simulink library "Electrical_to_Thermal_gen"  (R2016a)
settings: Solver=ode1  StartTime=0.0  StopTime=Inf  FixedStep=0.001  RelTol=1e-3
undefined symbols (not defined in the file): brakeresistors_Brc_Coolent_Inlet_Temp, brakeresistors_BRC_InvStError, brakeresistors_Brc_Powerderating, brakeresistors_BRCMaxPwr, brakeresistors_NumBrkResistors, Brc_Coolent_Inlet_Temp, BRC_InvStError, Brc_Powerderating, drvEmot_InvStEnable, drvEmot_InvStError, drvEmot_InvStInit, drvEmot_InvStReady, InvStEnable, InvStError, InvStInit, InvStReady, NumBrkResistors
libraries: simulink x3, Electrical_to_Thermal_gen x1
settings Model: Creator=SAHOPRA  LastModifiedBy=krishs1
settings DataIOCC: LimitDataPoints=on  SaveFormat=Array
settings OptimizationCC: BlockReduction=off  OptimizeBlockIOStorage=off  BufferReuse=off  GlobalBufferReuse=off  ExpressionFolding=off  ExpressionDepthLimit=2147483647  LocalBlockOutputs=off
settings DebuggingCC: UnderspecifiedInitializationDetection=Classic  MergeDetectMultiDrivingBlocksExec=none  SolverPrmCheckMsg=warning  StateNameClashWarn=warning
settings HardwareCC: ProdBitPerPointer=32  ProdLargestAtomicFloat=None  ProdIntDivRoundTo=Undefined  ProdEndianess=Unspecified  ProdWordSize=32  ProdHWDeviceType=32-bit Generic
settings ModelReferenceCC: PropagateSignalLabelsOutOfModel=off
settings RTWCC: SystemTargetFile=rti1005.tlc  MakeCommand=make_rti  TemplateMakefile=rti1005.tmf  Description=dSPACE DS1005 Hardware Platform
settings STFCustomTargetCC: ModelReferenceCompliant=off  GeneratePreprocessorConditionals=Disable all  CombineOutputUpdateFcns=on  MatFileLogging=on  MATLABClassNameForMDSCustomization=Simulink.SoftwareTarget.TargetSpecificTriggerConfigurationBase  CPPClassGenCompliant=on  GRTInterface=off  SystemTargetFile=rti1005.tlc
settings ConfigComp: CovModelRefEnable=Off

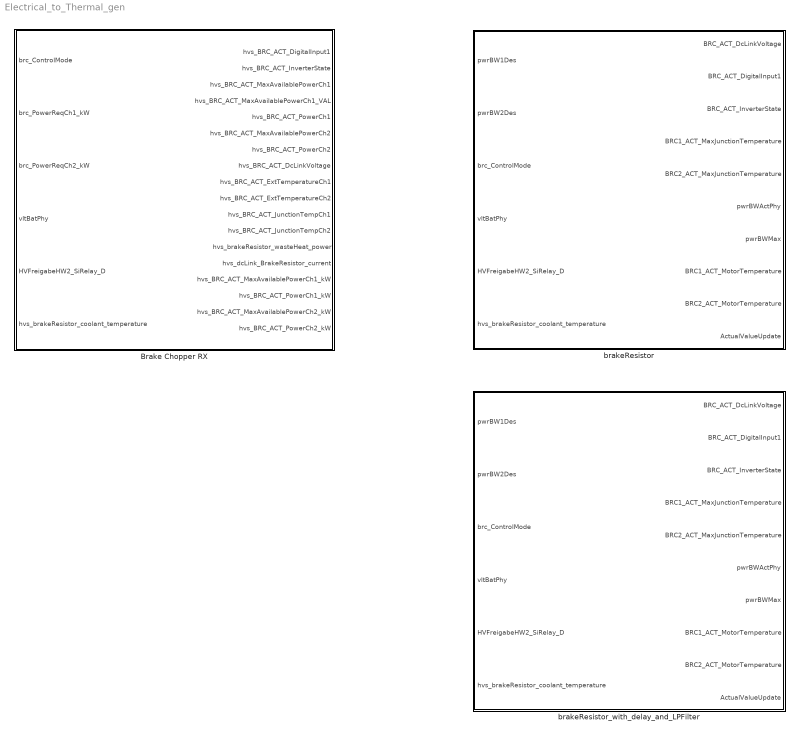
== system Electrical_to_Thermal_gen ==
  Brake Chopper RX : Subsystem
  brakeResistor : Subsystem
  brakeResistor_with_delay_and_LPFilter : Subsystem

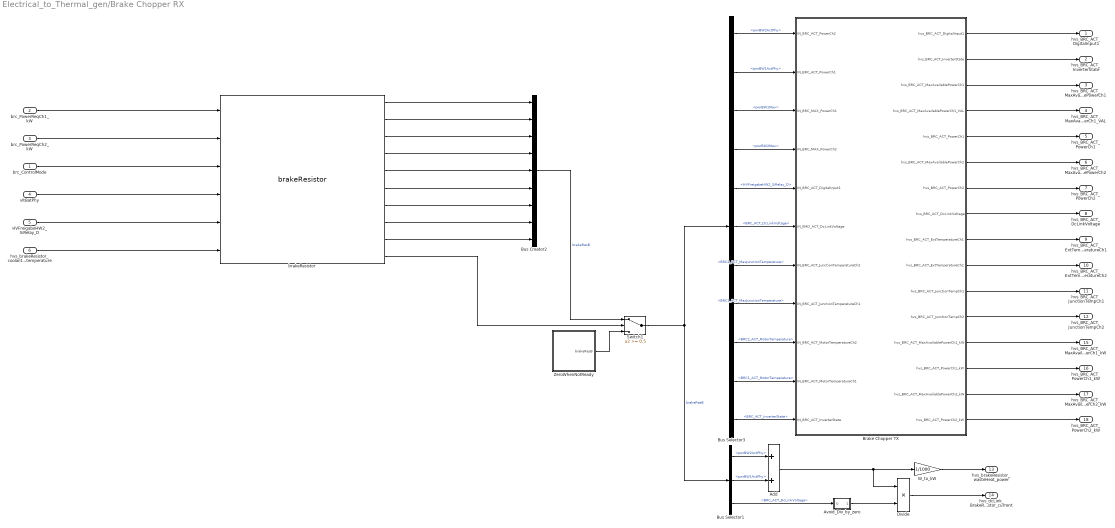
== system Electrical_to_Thermal_gen/Brake Chopper RX ==
  brc_ControlMode : Inport
  brc_PowerReqCh1_kW : Inport  Port=2
  brc_PowerReqCh2_kW : Inport  Port=3
  vltBatPhy : Inport  Port=4
  HVFreigabeHW2_SiRelay_D : Inport  Port=5
  hvs_brakeResistor_coolant_temperature : Inport  Port=6
  Add : Sum
  Avoid_Div_by_zero : Subsystem
  Brake Chopper TX : Subsystem
  Bus Creator2 : BusCreator  Inputs=9
  Bus Selector1 : BusSelector  OutputSignals=pwrBWActPhy.pwrBW2ActPhy,pwrBWActPhy.pwrBW1ActPhy,BRC_ACT_DcLinkVoltage
  Bus Selector3 : BusSelector  OutputSignals=pwrBWActPhy.pwrBW2ActPhy,pwrBWActPhy.pwrBW1ActPhy,pwrBWMax.pwrBW1Max,pwrBWMax.pwrBW2Max,HVFreigabeHW2_SiRelay_D,BRC_ACT_DcLinkVoltage,BRC2_ACT_MaxJunctionTemperature,BRC1_ACT_MaxJunctionTemperature,BRC2_ACT_MotorTemperature,BRC1_ACT_MotorTemperature,BRC_ACT_InverterState
  Divide : Product  Inputs=**
  Switch1 : Switch  Threshold=0.5
  W_to_kW : Gain  Gain=1/1000
      settings: AttributesFormatString=%<Description>
  ZeroWhenNotReady : Subsystem  TreatAsAtomicUnit=on
  brakeResistor : Electrical_to_Thermal_gen/brakeResistor  SystemSampleTime=-1
  hvs_BRC_ACT_DigitalInput1 : Outport
  hvs_BRC_ACT_InverterState : Outport  Port=2
  hvs_BRC_ACT_MaxAvailablePowerCh1 : Outport  Port=3
  hvs_BRC_ACT_MaxAvailablePowerCh1_VAL : Outport  Port=4
  hvs_BRC_ACT_PowerCh1 : Outport  Port=5
  hvs_BRC_ACT_MaxAvailablePowerCh2 : Outport  Port=6
  hvs_BRC_ACT_PowerCh2 : Outport  Port=7
  hvs_BRC_ACT_DcLinkVoltage : Outport  Port=8
  hvs_BRC_ACT_ExtTemperatureCh1 : Outport  Port=9
  hvs_BRC_ACT_ExtTemperatureCh2 : Outport  Port=10
  hvs_BRC_ACT_JunctionTempCh1 : Outport  Port=11
  hvs_BRC_ACT_JunctionTempCh2 : Outport  Port=12
  hvs_brakeResistor_wasteHeat_power : Outport  Port=13
  hvs_dcLink_BrakeResistor_current : Outport  Port=14
  hvs_BRC_ACT_MaxAvailablePowerCh1_kW : Outport  Port=15
  hvs_BRC_ACT_PowerCh1_kW : Outport  Port=16
  hvs_BRC_ACT_MaxAvailablePowerCh2_kW : Outport  Port=17
  hvs_BRC_ACT_PowerCh2_kW : Outport  Port=18
  wires:
  W_to_kW/1 -> hvs_brakeResistor_wasteHeat_power/1
  hvs_brakeResistor_coolant_temperature/1 -> brakeResistor/6
  Divide/1 -> hvs_dcLink_BrakeResistor_current/1
  Avoid_Div_by_zero/1(1/U) -> Divide/2
  Bus Selector1/3 -> Avoid_Div_by_zero/1(U)  "<BRC_ACT_DcLinkVoltage>"
  Add/1 -> W_to_kW/1, Divide/1
  Bus Selector1/2 -> Add/2  "<pwrBW1ActPhy>"
  Bus Selector1/1 -> Add/1  "<pwrBW2ActPhy>"
  HVFreigabeHW2_SiRelay_D/1 -> brakeResistor/5
  Brake Chopper TX/12(hvs_BRC_ACT_JunctionTempCh2) -> hvs_BRC_ACT_JunctionTempCh2/1
  Brake Chopper TX/11(hvs_BRC_ACT_JunctionTempCh1) -> hvs_BRC_ACT_JunctionTempCh1/1
  Brake Chopper TX/10(hvs_BRC_ACT_ExtTemperatureCh2) -> hvs_BRC_ACT_ExtTemperatureCh2/1
  Brake Chopper TX/9(hvs_BRC_ACT_ExtTemperatureCh1) -> hvs_BRC_ACT_ExtTemperatureCh1/1
  Brake Chopper TX/8(hvs_BRC_ACT_DcLinkVoltage) -> hvs_BRC_ACT_DcLinkVoltage/1
  Brake Chopper TX/7(hvs_BRC_ACT_PowerCh2) -> hvs_BRC_ACT_PowerCh2/1
  Brake Chopper TX/6(hvs_BRC_ACT_MaxAvailablePowerCh2) -> hvs_BRC_ACT_MaxAvailablePowerCh2/1
  Brake Chopper TX/5(hvs_BRC_ACT_PowerCh1) -> hvs_BRC_ACT_PowerCh1/1
  Brake Chopper TX/4(hvs_BRC_ACT_MaxAvailablePowerCh1_VAL) -> hvs_BRC_ACT_MaxAvailablePowerCh1_VAL/1
  Brake Chopper TX/3(hvs_BRC_ACT_MaxAvailablePowerCh1) -> hvs_BRC_ACT_MaxAvailablePowerCh1/1
  Brake Chopper TX/2(hvs_BRC_ACT_InverterState) -> hvs_BRC_ACT_InverterState/1
  Brake Chopper TX/1(hvs_BRC_ACT_DigitalInput1) -> hvs_BRC_ACT_DigitalInput1/1
  Bus Selector3/3 -> Brake Chopper TX/3(IN_BRC_MAX_PowerCh1)  "<pwrBW1Max>"
  Bus Selector3/5 -> Brake Chopper TX/5(IN_BRC_ACT_DigitalInput1)  "<HVFreigabeHW2_SiRelay_D>"
  Bus Selector3/4 -> Brake Chopper TX/4(IN_BRC_MAX_PowerCh2)  "<pwrBW2Max>"
  Bus Selector3/1 -> Brake Chopper TX/1(IN_BRC_ACT_PowerCh2)  "<pwrBW2ActPhy>"
  Bus Selector3/2 -> Brake Chopper TX/2(IN_BRC_ACT_PowerCh1)  "<pwrBW1ActPhy>"
  Bus Selector3/6 -> Brake Chopper TX/6(IN_EMD_ACT_DcLinkVoltage)  "<BRC_ACT_DcLinkVoltage>"
  Bus Selector3/7 -> Brake Chopper TX/7(IN_BRC_ACT_JunctionTemperatureCh2)  "<BRC2_ACT_MaxJunctionTemperature>"
  Bus Selector3/8 -> Brake Chopper TX/8(IN_BRC_ACT_JunctionTemperatureCh1)  "<BRC1_ACT_MaxJunctionTemperature>"
  Bus Selector3/9 -> Brake Chopper TX/9(IN_BRC_ACT_MotorTemperatureCh2)  "<BRC2_ACT_MotorTemperature>"
  Bus Selector3/10 -> Brake Chopper TX/10(IN_BRC_ACT_MotorTemperatureCh1)  "<BRC1_ACT_MotorTemperature>"
  Bus Selector3/11 -> Brake Chopper TX/11(IN_BRC_ACT_InverterState)  "<BRC_ACT_InverterState>"
  vltBatPhy/1 -> brakeResistor/4
  brc_PowerReqCh2_kW/1 -> brakeResistor/2
  brc_PowerReqCh1_kW/1 -> brakeResistor/1
  brc_ControlMode/1 -> brakeResistor/3
  Bus Creator2/1 -> Switch1/1  "brakeResB"
  Switch1/1 -> Bus Selector3/1, Bus Selector1/1  "brakeResB"
  ZeroWhenNotReady/1(brakeResB) -> Switch1/3
  brakeResistor/6 -> Bus Creator2/6
  brakeResistor/7 -> Bus Creator2/7
  brakeResistor/8 -> Bus Creator2/8
  brakeResistor/5 -> Bus Creator2/5
  brakeResistor/4 -> Bus Creator2/4
  brakeResistor/3 -> Bus Creator2/3
  brakeResistor/2 -> Bus Creator2/2
  brakeResistor/1 -> Bus Creator2/1
  brakeResistor/9 -> Bus Creator2/9
  Brake Chopper TX/13(hvs_BRC_ACT_MaxAvailablePowerCh1_kW) -> hvs_BRC_ACT_MaxAvailablePowerCh1_kW/1
  Brake Chopper TX/14(hvs_BRC_ACT_PowerCh1_kW) -> hvs_BRC_ACT_PowerCh1_kW/1
  Brake Chopper TX/15(hvs_BRC_ACT_MaxAvailablePowerCh2_kW) -> hvs_BRC_ACT_MaxAvailablePowerCh2_kW/1
  Brake Chopper TX/16(hvs_BRC_ACT_PowerCh2_kW) -> hvs_BRC_ACT_PowerCh2_kW/1
  brakeResistor/10 -> Switch1/2

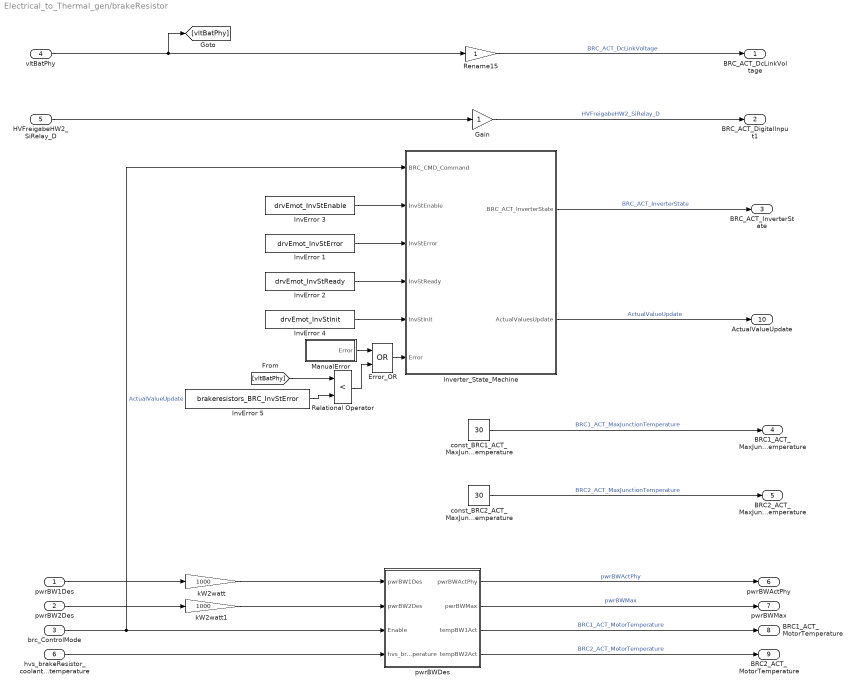
== system Electrical_to_Thermal_gen/brakeResistor ==
  pwrBW1Des : Inport
  pwrBW2Des : Inport  Port=2
  brc_ControlMode : Inport  Port=3
  vltBatPhy : Inport  Port=4
  HVFreigabeHW2_SiRelay_D : Inport  Port=5
  hvs_brakeResistor_coolant_temperature : Inport  Port=6
  Error_OR : Logic  Operator=OR  AllPortsSameDT=off  OutDataTypeStr=boolean
  Gain : Gain
  InvError 1 : Constant  Value=drvEmot_InvStError
  InvError 2 : Constant  Value=drvEmot_InvStReady
  InvError 3 : Constant  Value=drvEmot_InvStEnable
  InvError 4 : Constant  Value=drvEmot_InvStInit
  InvError 5 : Constant  Value=brakeresistors_BRC_InvStError
  Inverter_State_Machine : Stateflow chart  TreatAsAtomicUnit=on
  ManualError : Subsystem  TreatAsAtomicUnit=on
  Relational Operator : RelationalOperator  Operator=<  OutDataTypeStr=boolean
  Rename15 : Gain
  const_BRC1_ACT_MaxJunctionTemperature : Constant  Value=30
  const_BRC2_ACT_MaxJunctionTemperature : Constant  Value=30
  kW2watt : Gain  Gain=1000
  kW2watt1 : Gain  Gain=1000
  "pwrBWDes " : Subsystem
  BRC_ACT_DcLinkVoltage : Outport
  " BRC_ACT_DigitalInput1" : Outport  Port=2
  BRC_ACT_InverterState : Outport  Port=3
  BRC1_ACT_MaxJunctionTemperature : Outport  Port=4
  BRC2_ACT_MaxJunctionTemperature : Outport  Port=5
  pwrBWActPhy : Outport  Port=6
  pwrBWMax : Outport  Port=7
  BRC1_ACT_MotorTemperature : Outport  Port=8
  BRC2_ACT_MotorTemperature : Outport  Port=9
  ActualValueUpdate : Outport  Port=10
  wires:
  kW2watt1/1 -> "pwrBWDes "/2(pwrBW2Des)
  kW2watt/1 -> "pwrBWDes "/1(pwrBW1Des)
  pwrBW2Des/1 -> kW2watt1/1
  pwrBW1Des/1 -> kW2watt/1
  HVFreigabeHW2_SiRelay_D/1 -> Gain/1
  brc_ControlMode/1 -> "pwrBWDes "/3(Enable), Inverter_State_Machine/1(BRC_CMD_Command)  "ActualValueUpdate"
  Rename15/1 -> BRC_ACT_DcLinkVoltage/1  "BRC_ACT_DcLinkVoltage"
  "pwrBWDes "/4(tempBW2Act) -> BRC2_ACT_MotorTemperature/1  "BRC2_ACT_MotorTemperature"
  "pwrBWDes "/3(tempBW1Act) -> BRC1_ACT_MotorTemperature/1  "BRC1_ACT_MotorTemperature"
  Gain/1 -> " BRC_ACT_DigitalInput1"/1  "HVFreigabeHW2_SiRelay_D"
  const_BRC2_ACT_MaxJunctionTemperature/1 -> BRC2_ACT_MaxJunctionTemperature/1  "BRC2_ACT_MaxJunctionTemperature"
  const_BRC1_ACT_MaxJunctionTemperature/1 -> BRC1_ACT_MaxJunctionTemperature/1  "BRC1_ACT_MaxJunctionTemperature"
  "pwrBWDes "/2(pwrBWMax) -> pwrBWMax/1  "pwrBWMax"
  "pwrBWDes "/1(pwrBWActPhy) -> pwrBWActPhy/1  "pwrBWActPhy"
  hvs_brakeResistor_coolant_temperature/1 -> "pwrBWDes "/4(hvs_brakeResistor_coolant_temperature)
  InvError 1/1 -> Inverter_State_Machine/3(InvStError)
  InvError 2/1 -> Inverter_State_Machine/4(InvStReady)
  InvError 3/1 -> Inverter_State_Machine/2(InvStEnable)
  InvError 4/1 -> Inverter_State_Machine/5(InvStInit)
  Inverter_State_Machine/1(BRC_ACT_InverterState) -> BRC_ACT_InverterState/1  "BRC_ACT_InverterState"
  Error_OR/1 -> Inverter_State_Machine/6(Error)
  Inverter_State_Machine/2(ActualValuesUpdate) -> ActualValueUpdate/1  "ActualValueUpdate"
  ManualError/1(Error) -> Error_OR/1
  Relational Operator/1 -> Error_OR/2
  InvError 5/1 -> Relational Operator/2
  vltBatPhy/1 -> [vltBatPhy], Rename15/1
  [vltBatPhy] -> Relational Operator/1

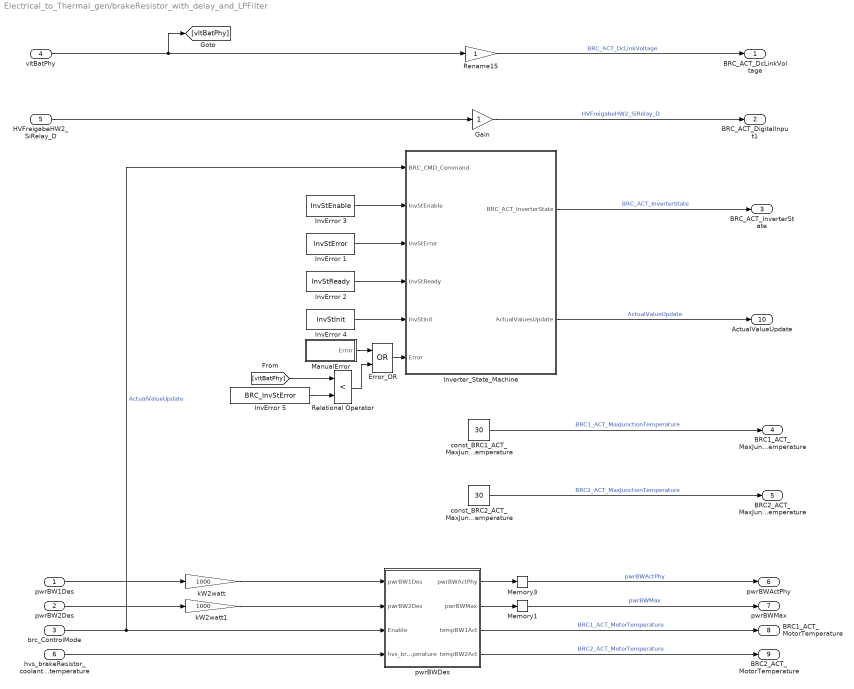
== system Electrical_to_Thermal_gen/brakeResistor_with_delay_and_LPFilter ==
  pwrBW1Des : Inport
  pwrBW2Des : Inport  Port=2
  brc_ControlMode : Inport  Port=3
  vltBatPhy : Inport  Port=4
  HVFreigabeHW2_SiRelay_D : Inport  Port=5
  hvs_brakeResistor_coolant_temperature : Inport  Port=6
  Error_OR : Logic  Operator=OR  AllPortsSameDT=off  OutDataTypeStr=boolean
  Gain : Gain
  InvError 1 : Constant  Value=InvStError
  InvError 2 : Constant  Value=InvStReady
  InvError 3 : Constant  Value=InvStEnable
  InvError 4 : Constant  Value=InvStInit
  InvError 5 : Constant  Value=BRC_InvStError
  Inverter_State_Machine : Stateflow chart  TreatAsAtomicUnit=on
  ManualError : Subsystem  TreatAsAtomicUnit=on
  Memory1 : Memory
  Memory3 : Memory
  Relational Operator : RelationalOperator  Operator=<  OutDataTypeStr=boolean
  Rename15 : Gain
  const_BRC1_ACT_MaxJunctionTemperature : Constant  Value=30
  const_BRC2_ACT_MaxJunctionTemperature : Constant  Value=30
  kW2watt : Gain  Gain=1000
  kW2watt1 : Gain  Gain=1000
  "pwrBWDes " : Subsystem
  BRC_ACT_DcLinkVoltage : Outport
  " BRC_ACT_DigitalInput1" : Outport  Port=2
  BRC_ACT_InverterState : Outport  Port=3
  BRC1_ACT_MaxJunctionTemperature : Outport  Port=4
  BRC2_ACT_MaxJunctionTemperature : Outport  Port=5
  pwrBWActPhy : Outport  Port=6
  pwrBWMax : Outport  Port=7
  BRC1_ACT_MotorTemperature : Outport  Port=8
  BRC2_ACT_MotorTemperature : Outport  Port=9
  ActualValueUpdate : Outport  Port=10
  wires:
  kW2watt1/1 -> "pwrBWDes "/2(pwrBW2Des)
  kW2watt/1 -> "pwrBWDes "/1(pwrBW1Des)
  pwrBW2Des/1 -> kW2watt1/1
  pwrBW1Des/1 -> kW2watt/1
  HVFreigabeHW2_SiRelay_D/1 -> Gain/1
  brc_ControlMode/1 -> "pwrBWDes "/3(Enable), Inverter_State_Machine/1(BRC_CMD_Command)  "ActualValueUpdate"
  Rename15/1 -> BRC_ACT_DcLinkVoltage/1  "BRC_ACT_DcLinkVoltage"
  "pwrBWDes "/4(tempBW2Act) -> BRC2_ACT_MotorTemperature/1  "BRC2_ACT_MotorTemperature"
  "pwrBWDes "/3(tempBW1Act) -> BRC1_ACT_MotorTemperature/1  "BRC1_ACT_MotorTemperature"
  Gain/1 -> " BRC_ACT_DigitalInput1"/1  "HVFreigabeHW2_SiRelay_D"
  const_BRC2_ACT_MaxJunctionTemperature/1 -> BRC2_ACT_MaxJunctionTemperature/1  "BRC2_ACT_MaxJunctionTemperature"
  const_BRC1_ACT_MaxJunctionTemperature/1 -> BRC1_ACT_MaxJunctionTemperature/1  "BRC1_ACT_MaxJunctionTemperature"
  Memory1/1 -> pwrBWMax/1  "pwrBWMax"
  "pwrBWDes "/2(pwrBWMax) -> Memory1/1
  Memory3/1 -> pwrBWActPhy/1  "pwrBWActPhy"
  "pwrBWDes "/1(pwrBWActPhy) -> Memory3/1
  hvs_brakeResistor_coolant_temperature/1 -> "pwrBWDes "/4(hvs_brakeResistor_coolant_temperature)
  InvError 1/1 -> Inverter_State_Machine/3(InvStError)
  InvError 2/1 -> Inverter_State_Machine/4(InvStReady)
  InvError 3/1 -> Inverter_State_Machine/2(InvStEnable)
  InvError 4/1 -> Inverter_State_Machine/5(InvStInit)
  Inverter_State_Machine/1(BRC_ACT_InverterState) -> BRC_ACT_InverterState/1  "BRC_ACT_InverterState"
  Error_OR/1 -> Inverter_State_Machine/6(Error)
  Inverter_State_Machine/2(ActualValuesUpdate) -> ActualValueUpdate/1  "ActualValueUpdate"
  ManualError/1(Error) -> Error_OR/1
  Relational Operator/1 -> Error_OR/2
  InvError 5/1 -> Relational Operator/2
  vltBatPhy/1 -> [vltBatPhy], Rename15/1
  [vltBatPhy] -> Relational Operator/1

== system Electrical_to_Thermal_gen/Brake Chopper RX/Avoid_Div_by_zero ==
  U : Inport
  Constant : Constant  Value=10^-6
  Divide : Product  Inputs=/*
  Math Function : Math  Operator=square  SaturateOnIntegerOverflow=on
  Sum : Sum  Inputs=++|
  1/U : Outport
  wires:
  U/1 -> Sum/2
  Constant/1 -> Sum/1
  Sum/1 -> Math Function/1, Divide/2
  Math Function/1 -> Divide/1
  Divide/1 -> 1/U/1

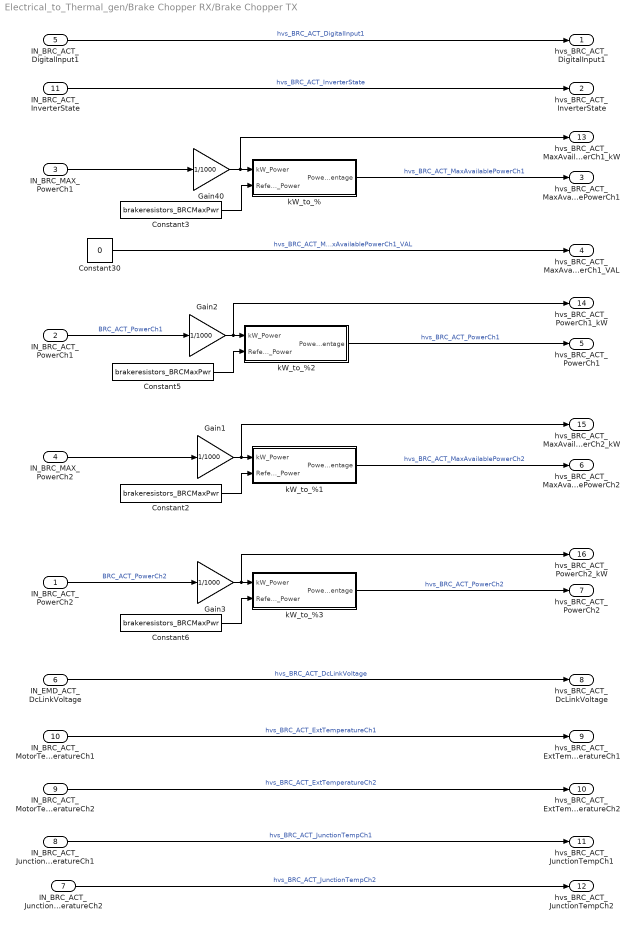
== system Electrical_to_Thermal_gen/Brake Chopper RX/Brake Chopper TX ==
  IN_BRC_ACT_PowerCh2 : Inport
  IN_BRC_ACT_PowerCh1 : Inport  Port=2
  IN_BRC_MAX_PowerCh1 : Inport  Port=3
  IN_BRC_MAX_PowerCh2 : Inport  Port=4
  IN_BRC_ACT_DigitalInput1 : Inport  Port=5
  IN_EMD_ACT_DcLinkVoltage : Inport  Port=6
  IN_BRC_ACT_JunctionTemperatureCh2 : Inport  Port=7
  IN_BRC_ACT_JunctionTemperatureCh1 : Inport  Port=8
  IN_BRC_ACT_MotorTemperatureCh2 : Inport  Port=9
  IN_BRC_ACT_MotorTemperatureCh1 : Inport  Port=10
  IN_BRC_ACT_InverterState : Inport  Port=11
  Constant{2..3,5..6} (4 alike) : Constant  Value=brakeresistors_BRCMaxPwr
  Constant30 : Constant  Value=0
  Gain{1..3,40} (4 alike) : Gain  Gain=1/1000
  kW_to_% : Subsystem
  kW_to_%1 : Subsystem
  kW_to_%2 : Subsystem
  kW_to_%3 : Subsystem
  hvs_BRC_ACT_DigitalInput1 : Outport
  hvs_BRC_ACT_InverterState : Outport  Port=2
  hvs_BRC_ACT_MaxAvailablePowerCh1 : Outport  Port=3
  hvs_BRC_ACT_MaxAvailablePowerCh1_VAL : Outport  Port=4
  hvs_BRC_ACT_PowerCh1 : Outport  Port=5
  hvs_BRC_ACT_MaxAvailablePowerCh2 : Outport  Port=6
  hvs_BRC_ACT_PowerCh2 : Outport  Port=7
  hvs_BRC_ACT_DcLinkVoltage : Outport  Port=8
  hvs_BRC_ACT_ExtTemperatureCh1 : Outport  Port=9
  hvs_BRC_ACT_ExtTemperatureCh2 : Outport  Port=10
  hvs_BRC_ACT_JunctionTempCh1 : Outport  Port=11
  hvs_BRC_ACT_JunctionTempCh2 : Outport  Port=12
  hvs_BRC_ACT_MaxAvailablePowerCh1_kW : Outport  Port=13
  hvs_BRC_ACT_PowerCh1_kW : Outport  Port=14
  hvs_BRC_ACT_MaxAvailablePowerCh2_kW : Outport  Port=15
  hvs_BRC_ACT_PowerCh2_kW : Outport  Port=16
  wires:
  Constant30/1 -> hvs_BRC_ACT_MaxAvailablePowerCh1_VAL/1  "hvs_BRC_ACT_MaxAvailablePowerCh1_VAL"
  Constant6/1 -> kW_to_%3/2(Reference_Power)
  Gain3/1 -> hvs_BRC_ACT_PowerCh2_kW/1, kW_to_%3/1(kW_Power)
  IN_BRC_ACT_PowerCh2/1 -> Gain3/1  "BRC_ACT_PowerCh2"
  Constant5/1 -> kW_to_%2/2(Reference_Power)
  Gain2/1 -> hvs_BRC_ACT_PowerCh1_kW/1, kW_to_%2/1(kW_Power)
  IN_BRC_ACT_PowerCh1/1 -> Gain2/1  "BRC_ACT_PowerCh1"
  Gain1/1 -> hvs_BRC_ACT_MaxAvailablePowerCh2_kW/1, kW_to_%1/1(kW_Power)
  Constant2/1 -> kW_to_%1/2(Reference_Power)
  Constant3/1 -> kW_to_%/2(Reference_Power)
  Gain40/1 -> hvs_BRC_ACT_MaxAvailablePowerCh1_kW/1, kW_to_%/1(kW_Power)
  kW_to_%1/1(Power_Percentage) -> hvs_BRC_ACT_MaxAvailablePowerCh2/1  "hvs_BRC_ACT_MaxAvailablePowerCh2"
  IN_BRC_MAX_PowerCh2/1 -> Gain1/1
  kW_to_%/1(Power_Percentage) -> hvs_BRC_ACT_MaxAvailablePowerCh1/1  "hvs_BRC_ACT_MaxAvailablePowerCh1"
  IN_BRC_MAX_PowerCh1/1 -> Gain40/1
  IN_BRC_ACT_DigitalInput1/1 -> hvs_BRC_ACT_DigitalInput1/1  "hvs_BRC_ACT_DigitalInput1"
  IN_BRC_ACT_JunctionTemperatureCh1/1 -> hvs_BRC_ACT_JunctionTempCh1/1  "hvs_BRC_ACT_JunctionTempCh1"
  IN_BRC_ACT_JunctionTemperatureCh2/1 -> hvs_BRC_ACT_JunctionTempCh2/1  "hvs_BRC_ACT_JunctionTempCh2"
  IN_EMD_ACT_DcLinkVoltage/1 -> hvs_BRC_ACT_DcLinkVoltage/1  "hvs_BRC_ACT_DcLinkVoltage"
  kW_to_%3/1(Power_Percentage) -> hvs_BRC_ACT_PowerCh2/1  "hvs_BRC_ACT_PowerCh2"
  IN_BRC_ACT_MotorTemperatureCh2/1 -> hvs_BRC_ACT_ExtTemperatureCh2/1  "hvs_BRC_ACT_ExtTemperatureCh2"
  kW_to_%2/1(Power_Percentage) -> hvs_BRC_ACT_PowerCh1/1  "hvs_BRC_ACT_PowerCh1"
  IN_BRC_ACT_MotorTemperatureCh1/1 -> hvs_BRC_ACT_ExtTemperatureCh1/1  "hvs_BRC_ACT_ExtTemperatureCh1"
  IN_BRC_ACT_InverterState/1 -> hvs_BRC_ACT_InverterState/1  "hvs_BRC_ACT_InverterState"

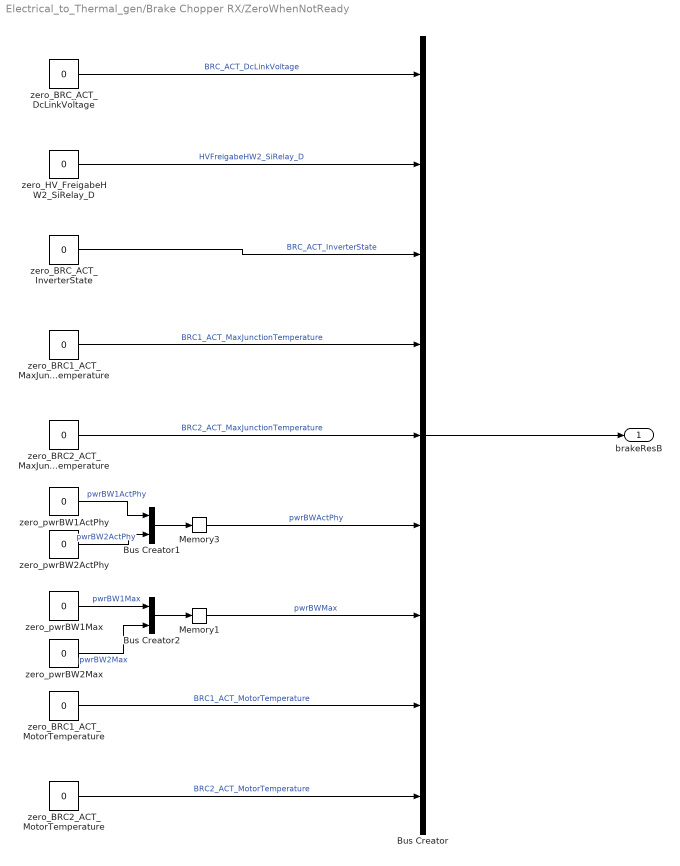
== system Electrical_to_Thermal_gen/Brake Chopper RX/ZeroWhenNotReady ==
  Bus Creator : BusCreator  Inputs=9
  Bus Creator1 : BusCreator  Inputs=2
  Bus Creator2 : BusCreator  Inputs=2
  Memory1 : Memory  InheritSampleTime=on
  Memory3 : Memory  InheritSampleTime=on
  zero_BRC1_ACT_MaxJunctionTemperature : Constant  Value=0
  zero_BRC1_ACT_MotorTemperature : Constant  Value=0
  zero_BRC2_ACT_MaxJunctionTemperature : Constant  Value=0
  zero_BRC2_ACT_MotorTemperature : Constant  Value=0
  zero_BRC_ACT_DcLinkVoltage : Constant  Value=0
  zero_BRC_ACT_InverterState : Constant  Value=0
  zero_HV_FreigabeHW2_SiRelay_D : Constant  Value=0
  zero_pwrBW1ActPhy : Constant  Value=0
  zero_pwrBW1Max : Constant  Value=0
  zero_pwrBW2ActPhy : Constant  Value=0
  zero_pwrBW2Max : Constant  Value=0
  brakeResB : Outport
  wires:
  zero_HV_FreigabeHW2_SiRelay_D/1 -> Bus Creator/2  "HVFreigabeHW2_SiRelay_D"
  zero_BRC_ACT_InverterState/1 -> Bus Creator/3  "BRC_ACT_InverterState"
  zero_BRC1_ACT_MaxJunctionTemperature/1 -> Bus Creator/4  "BRC1_ACT_MaxJunctionTemperature"
  zero_BRC2_ACT_MaxJunctionTemperature/1 -> Bus Creator/5  "BRC2_ACT_MaxJunctionTemperature"
  Memory3/1 -> Bus Creator/6  "pwrBWActPhy"
  Memory1/1 -> Bus Creator/7  "pwrBWMax"
  Bus Creator1/1 -> Memory3/1
  zero_pwrBW1ActPhy/1 -> Bus Creator1/1  "pwrBW1ActPhy"
  zero_pwrBW2ActPhy/1 -> Bus Creator1/2  "pwrBW2ActPhy"
  Bus Creator2/1 -> Memory1/1
  zero_pwrBW1Max/1 -> Bus Creator2/1  "pwrBW1Max"
  zero_pwrBW2Max/1 -> Bus Creator2/2  "pwrBW2Max"
  Bus Creator/1 -> brakeResB/1
  zero_BRC_ACT_DcLinkVoltage/1 -> Bus Creator/1  "BRC_ACT_DcLinkVoltage"
  zero_BRC2_ACT_MotorTemperature/1 -> Bus Creator/9  "BRC2_ACT_MotorTemperature"
  zero_BRC1_ACT_MotorTemperature/1 -> Bus Creator/8  "BRC1_ACT_MotorTemperature"

== system Electrical_to_Thermal_gen/brakeResistor/ManualError ==
  ErrorSwitch : ManualSwitch
  InvError : Constant
  NoError : Constant  Value=0
  Error : Outport
  wires:
  NoError/1 -> ErrorSwitch/1
  InvError/1 -> ErrorSwitch/2
  ErrorSwitch/1 -> Error/1

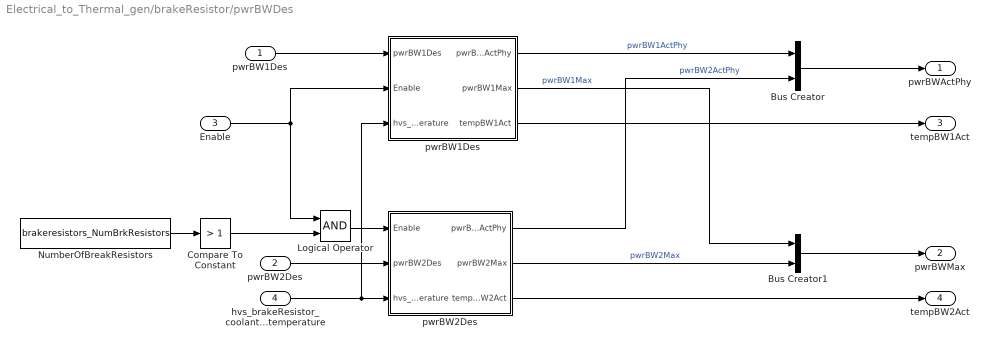
== system Electrical_to_Thermal_gen/brakeResistor/pwrBWDes  ==
  pwrBW1Des : Inport
  pwrBW2Des : Inport  Port=2
  Enable : Inport  Port=3
  hvs_brakeResistor_coolant_temperature : Inport  Port=4
  Bus Creator : BusCreator  Inputs=2
  Bus Creator1 : BusCreator  Inputs=2
  Compare To Constant : simulink/Logic and Bit Operations/Compare To Constant  relop=>  const=1  OutDataTypeStr=boolean
  Logical Operator : Logic  AllPortsSameDT=off  OutDataTypeStr=boolean
  NumberOfBreakResistors : Constant  Value=brakeresistors_NumBrkResistors
  "pwrBW1Des " : Subsystem
  "pwrBW2Des " : Subsystem
  pwrBWActPhy : Outport
  pwrBWMax : Outport  Port=2
  tempBW1Act : Outport  Port=3
  tempBW2Act : Outport  Port=4
  wires:
  hvs_brakeResistor_coolant_temperature/1 -> "pwrBW1Des "/3(hvs_brakeResistor_coolant_temperature), "pwrBW2Des "/3(hvs_brakeResistor_coolant_temperature)
  "pwrBW2Des "/3(tempBW2Act) -> tempBW2Act/1
  "pwrBW1Des "/3(tempBW1Act) -> tempBW1Act/1
  Enable/1 -> Logical Operator/1, "pwrBW1Des "/2(Enable)
  "pwrBW2Des "/2(pwrBW2Max) -> Bus Creator1/2  "pwrBW2Max"
  "pwrBW1Des "/2(pwrBW1Max) -> Bus Creator1/1  "pwrBW1Max"
  "pwrBW1Des "/1(pwrBW1ActPhy) -> Bus Creator/1  "pwrBW1ActPhy"
  Bus Creator1/1 -> pwrBWMax/1
  Bus Creator/1 -> pwrBWActPhy/1
  pwrBW2Des/1 -> "pwrBW2Des "/2(pwrBW2Des)
  pwrBW1Des/1 -> "pwrBW1Des "/1(pwrBW1Des)
  NumberOfBreakResistors/1 -> Compare To Constant/1
  Compare To Constant/1 -> Logical Operator/2
  Logical Operator/1 -> "pwrBW2Des "/1(Enable)
  "pwrBW2Des "/1(pwrBW2ActPhy) -> Bus Creator/2  "pwrBW2ActPhy"

== system Electrical_to_Thermal_gen/brakeResistor_with_delay_and_LPFilter/ManualError ==
  ErrorSwitch : ManualSwitch
  InvError : Constant
  NoError : Constant  Value=0
  Error : Outport
  wires:
  NoError/1 -> ErrorSwitch/1
  InvError/1 -> ErrorSwitch/2
  ErrorSwitch/1 -> Error/1

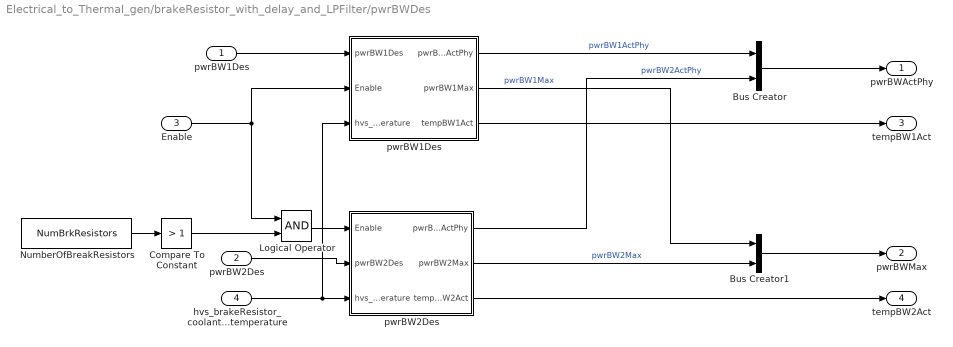
== system Electrical_to_Thermal_gen/brakeResistor_with_delay_and_LPFilter/pwrBWDes  ==
  pwrBW1Des : Inport
  pwrBW2Des : Inport  Port=2
  Enable : Inport  Port=3
  hvs_brakeResistor_coolant_temperature : Inport  Port=4
  Bus Creator : BusCreator  Inputs=2
  Bus Creator1 : BusCreator  Inputs=2
  Compare To Constant : simulink/Logic and Bit Operations/Compare To Constant  relop=>  const=1  OutDataTypeStr=boolean
  Logical Operator : Logic  AllPortsSameDT=off  OutDataTypeStr=boolean
  NumberOfBreakResistors : Constant  Value=NumBrkResistors
  "pwrBW1Des " : Subsystem
  "pwrBW2Des " : Subsystem
  pwrBWActPhy : Outport
  pwrBWMax : Outport  Port=2
  tempBW1Act : Outport  Port=3
  tempBW2Act : Outport  Port=4
  wires:
  hvs_brakeResistor_coolant_temperature/1 -> "pwrBW1Des "/3(hvs_brakeResistor_coolant_temperature), "pwrBW2Des "/3(hvs_brakeResistor_coolant_temperature)
  "pwrBW2Des "/3(tempBW2Act) -> tempBW2Act/1
  "pwrBW1Des "/3(tempBW1Act) -> tempBW1Act/1
  Enable/1 -> Logical Operator/1, "pwrBW1Des "/2(Enable)
  "pwrBW2Des "/2(pwrBW2Max) -> Bus Creator1/2  "pwrBW2Max"
  "pwrBW1Des "/2(pwrBW1Max) -> Bus Creator1/1  "pwrBW1Max"
  "pwrBW1Des "/1(pwrBW1ActPhy) -> Bus Creator/1  "pwrBW1ActPhy"
  Bus Creator1/1 -> pwrBWMax/1
  Bus Creator/1 -> pwrBWActPhy/1
  pwrBW2Des/1 -> "pwrBW2Des "/2(pwrBW2Des)
  pwrBW1Des/1 -> "pwrBW1Des "/1(pwrBW1Des)
  NumberOfBreakResistors/1 -> Compare To Constant/1
  Compare To Constant/1 -> Logical Operator/2
  Logical Operator/1 -> "pwrBW2Des "/1(Enable)
  "pwrBW2Des "/1(pwrBW2ActPhy) -> Bus Creator/2  "pwrBW2ActPhy"

== system Electrical_to_Thermal_gen/Brake Chopper RX/Brake Chopper TX/kW_to_% ==
  kW_Power : Inport
  Reference_Power : Inport  Port=2
  Constant : Constant  Value=100
  Divide1 : Product  Inputs=*/
  Product1 : Product  RndMeth=Zero
  Power_Percentage : Outport
  wires:
  Constant/1 -> Product1/2
  Divide1/1 -> Product1/1
  Reference_Power/1 -> Divide1/2  "Reference_Power"
  Product1/1 -> Power_Percentage/1  "Power_Percentage"
  kW_Power/1 -> Divide1/1  "kW_Power"

== system Electrical_to_Thermal_gen/Brake Chopper RX/Brake Chopper TX/kW_to_%1 ==
  kW_Power : Inport
  Reference_Power : Inport  Port=2
  Constant : Constant  Value=100
  Divide1 : Product  Inputs=*/
  Product1 : Product  RndMeth=Zero
  Power_Percentage : Outport
  wires:
  kW_Power/1 -> Divide1/1  "kW_Power"
  Product1/1 -> Power_Percentage/1  "Power_Percentage"
  Reference_Power/1 -> Divide1/2  "Reference_Power"
  Divide1/1 -> Product1/1
  Constant/1 -> Product1/2

== system Electrical_to_Thermal_gen/Brake Chopper RX/Brake Chopper TX/kW_to_%2 ==
  kW_Power : Inport
  Reference_Power : Inport  Port=2
  Constant : Constant  Value=100
  Divide1 : Product  Inputs=*/
  Product1 : Product  RndMeth=Zero
  Power_Percentage : Outport
  wires:
  Constant/1 -> Product1/2
  Divide1/1 -> Product1/1
  Reference_Power/1 -> Divide1/2  "Reference_Power"
  Product1/1 -> Power_Percentage/1  "Power_Percentage"
  kW_Power/1 -> Divide1/1  "kW_Power"

== system Electrical_to_Thermal_gen/Brake Chopper RX/Brake Chopper TX/kW_to_%3 ==
  kW_Power : Inport
  Reference_Power : Inport  Port=2
  Constant : Constant  Value=100
  Divide1 : Product  Inputs=*/
  Product1 : Product  RndMeth=Zero
  Power_Percentage : Outport
  wires:
  kW_Power/1 -> Divide1/1  "kW_Power"
  Product1/1 -> Power_Percentage/1  "Power_Percentage"
  Reference_Power/1 -> Divide1/2  "Reference_Power"
  Divide1/1 -> Product1/1
  Constant/1 -> Product1/2

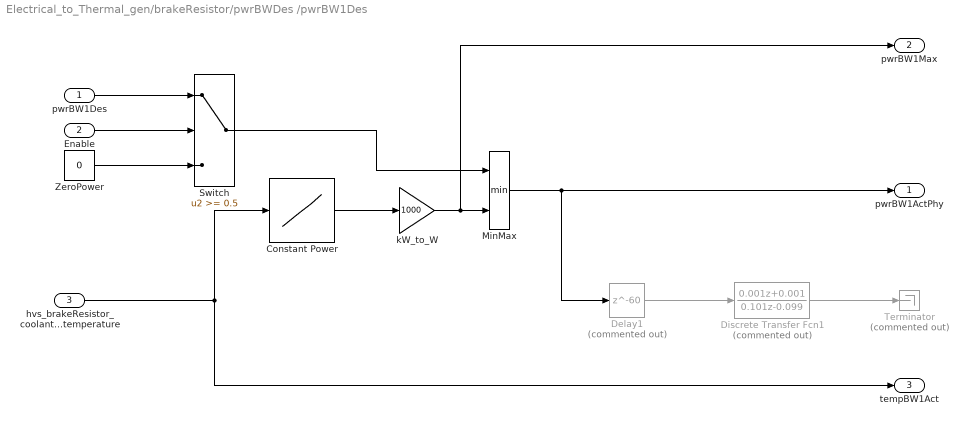
== system Electrical_to_Thermal_gen/brakeResistor/pwrBWDes /pwrBW1Des  ==
  pwrBW1Des : Inport
  Enable : Inport  Port=2
  hvs_brakeResistor_coolant_temperature : Inport  Port=3
  Constant Power : Lookup_n-D  NumberOfTableDimensions=1  BreakpointsForDimension1=brakeresistors_Brc_Coolent_Inlet_Temp  Table=brakeresistors_Brc_Powerderating  ExtrapMethod=Clip  UseLastTableValue=on  RndMeth=Simplest  InputSameDT=on
  Delay1 : Delay  Commented=on  DelayLength=60
  Discrete Transfer Fcn1 : DiscreteTransferFcn  Commented=on  Numerator=[0.001 0.001]  Denominator=[0.101 -0.099]
  MinMax : MinMax  Inputs=2
  Switch : Switch  Threshold=0.5
  Terminator : Terminator  Commented=on
  ZeroPower : Constant  Value=0
  kW_to_W : Gain  Gain=1000
  pwrBW1ActPhy : Outport
  pwrBW1Max : Outport  Port=2
  tempBW1Act : Outport  Port=3
  wires:
  hvs_brakeResistor_coolant_temperature/1 -> Constant Power/1, tempBW1Act/1
  Delay1/1 -> Discrete Transfer Fcn1/1
  MinMax/1 -> pwrBW1ActPhy/1, Delay1/1
  pwrBW1Des/1 -> Switch/1
  ZeroPower/1 -> Switch/3
  Switch/1 -> MinMax/1
  Enable/1 -> Switch/2
  Constant Power/1 -> kW_to_W/1
  Discrete Transfer Fcn1/1 -> Terminator/1
  kW_to_W/1 -> pwrBW1Max/1, MinMax/2

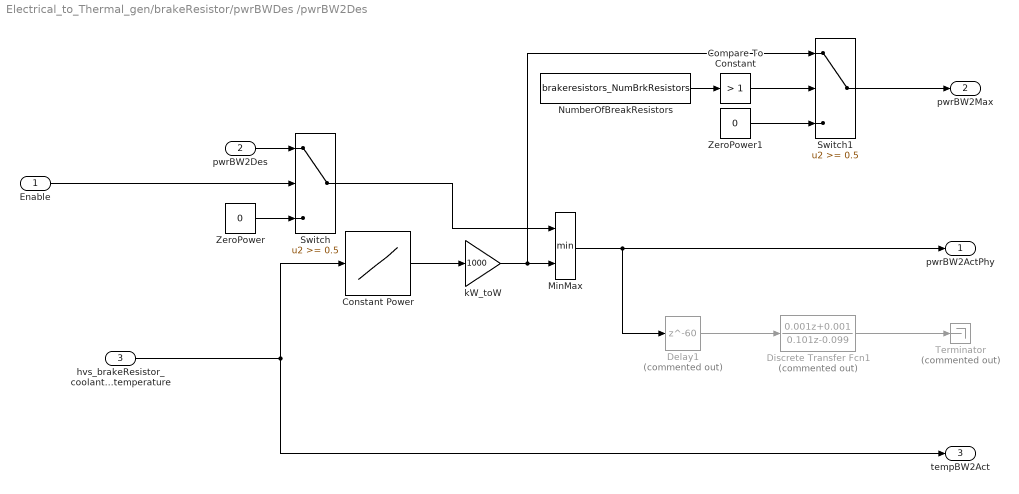
== system Electrical_to_Thermal_gen/brakeResistor/pwrBWDes /pwrBW2Des  ==
  Enable : Inport
  pwrBW2Des : Inport  Port=2
  hvs_brakeResistor_coolant_temperature : Inport  Port=3
  Compare To Constant : simulink/Logic and Bit Operations/Compare To Constant  relop=>  const=1  OutDataTypeStr=boolean
  Constant Power : Lookup_n-D  NumberOfTableDimensions=1  BreakpointsForDimension1=brakeresistors_Brc_Coolent_Inlet_Temp  Table=brakeresistors_Brc_Powerderating  ExtrapMethod=Clip  UseLastTableValue=on  RndMeth=Simplest  InputSameDT=on
  Delay1 : Delay  Commented=on  DelayLength=60
  Discrete Transfer Fcn1 : DiscreteTransferFcn  Commented=on  Numerator=[0.001 0.001]  Denominator=[0.101 -0.099]
  MinMax : MinMax  Inputs=2
  NumberOfBreakResistors : Constant  Value=brakeresistors_NumBrkResistors
  Switch : Switch  Threshold=0.5
  Switch1 : Switch  Threshold=0.5
  Terminator : Terminator  Commented=on
  ZeroPower : Constant  Value=0
  ZeroPower1 : Constant  Value=0
  kW_toW : Gain  Gain=1000
  pwrBW2ActPhy : Outport
  pwrBW2Max : Outport  Port=2
  tempBW2Act : Outport  Port=3
  wires:
  Enable/1 -> Switch/2
  Switch1/1 -> pwrBW2Max/1
  ZeroPower1/1 -> Switch1/3
  hvs_brakeResistor_coolant_temperature/1 -> Constant Power/1, tempBW2Act/1
  Discrete Transfer Fcn1/1 -> Terminator/1
  Delay1/1 -> Discrete Transfer Fcn1/1
  MinMax/1 -> pwrBW2ActPhy/1, Delay1/1
  kW_toW/1 -> MinMax/2, Switch1/1
  pwrBW2Des/1 -> Switch/1
  ZeroPower/1 -> Switch/3
  Switch/1 -> MinMax/1
  Constant Power/1 -> kW_toW/1
  NumberOfBreakResistors/1 -> Compare To Constant/1
  Compare To Constant/1 -> Switch1/2

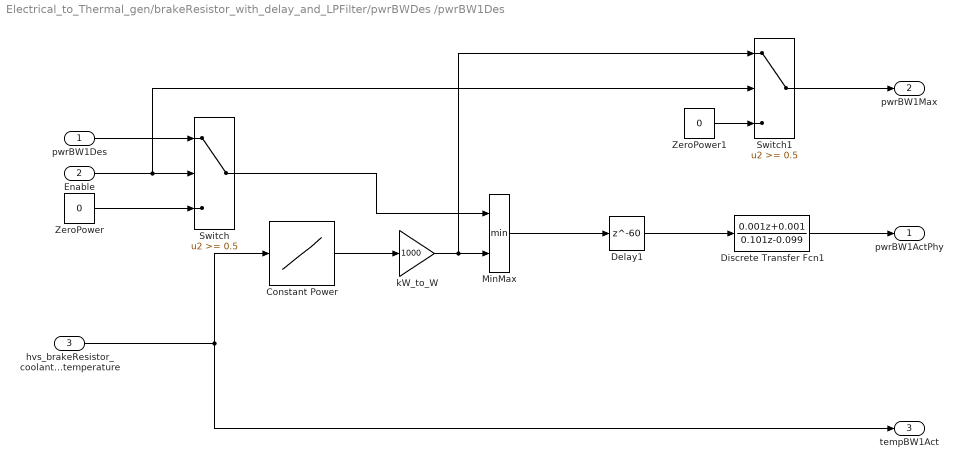
== system Electrical_to_Thermal_gen/brakeResistor_with_delay_and_LPFilter/pwrBWDes /pwrBW1Des  ==
  pwrBW1Des : Inport
  Enable : Inport  Port=2
  hvs_brakeResistor_coolant_temperature : Inport  Port=3
  Constant Power : Lookup_n-D  NumberOfTableDimensions=1  BreakpointsForDimension1=Brc_Coolent_Inlet_Temp  Table=Brc_Powerderating  ExtrapMethod=Clip  UseLastTableValue=on  RndMeth=Simplest  InputSameDT=on
  Delay1 : Delay  DelayLength=60
  Discrete Transfer Fcn1 : DiscreteTransferFcn  Numerator=[0.001 0.001]  Denominator=[0.101 -0.099]
  MinMax : MinMax  Inputs=2
  Switch : Switch  Threshold=0.5
  Switch1 : Switch  Threshold=0.5
  ZeroPower : Constant  Value=0
  ZeroPower1 : Constant  Value=0
  kW_to_W : Gain  Gain=1000
  pwrBW1ActPhy : Outport
  pwrBW1Max : Outport  Port=2
  tempBW1Act : Outport  Port=3
  wires:
  hvs_brakeResistor_coolant_temperature/1 -> Constant Power/1, tempBW1Act/1
  Delay1/1 -> Discrete Transfer Fcn1/1
  MinMax/1 -> Delay1/1
  pwrBW1Des/1 -> Switch/1
  kW_to_W/1 -> Switch1/1, MinMax/2
  ZeroPower/1 -> Switch/3
  Switch/1 -> MinMax/1
  Enable/1 -> Switch1/2, Switch/2
  Constant Power/1 -> kW_to_W/1
  ZeroPower1/1 -> Switch1/3
  Switch1/1 -> pwrBW1Max/1
  Discrete Transfer Fcn1/1 -> pwrBW1ActPhy/1

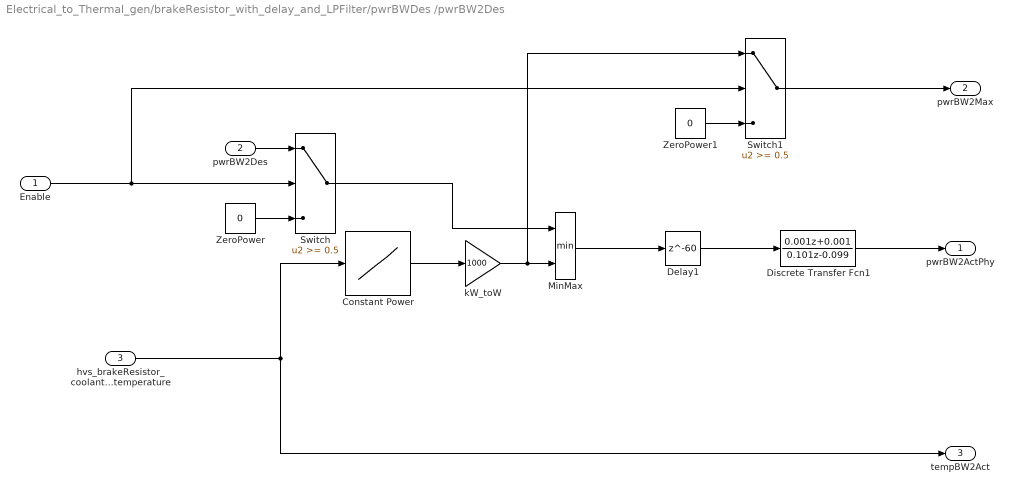
== system Electrical_to_Thermal_gen/brakeResistor_with_delay_and_LPFilter/pwrBWDes /pwrBW2Des  ==
  Enable : Inport
  pwrBW2Des : Inport  Port=2
  hvs_brakeResistor_coolant_temperature : Inport  Port=3
  Constant Power : Lookup_n-D  NumberOfTableDimensions=1  BreakpointsForDimension1=Brc_Coolent_Inlet_Temp  Table=Brc_Powerderating  ExtrapMethod=Clip  UseLastTableValue=on  RndMeth=Simplest  InputSameDT=on
  Delay1 : Delay  DelayLength=60
  Discrete Transfer Fcn1 : DiscreteTransferFcn  Numerator=[0.001 0.001]  Denominator=[0.101 -0.099]
  MinMax : MinMax  Inputs=2
  Switch : Switch  Threshold=0.5
  Switch1 : Switch  Threshold=0.5
  ZeroPower : Constant  Value=0
  ZeroPower1 : Constant  Value=0
  kW_toW : Gain  Gain=1000
  pwrBW2ActPhy : Outport
  pwrBW2Max : Outport  Port=2
  tempBW2Act : Outport  Port=3
  wires:
  Enable/1 -> Switch1/2, Switch/2
  Switch1/1 -> pwrBW2Max/1
  ZeroPower1/1 -> Switch1/3
  hvs_brakeResistor_coolant_temperature/1 -> Constant Power/1, tempBW2Act/1
  Delay1/1 -> Discrete Transfer Fcn1/1
  MinMax/1 -> Delay1/1
  kW_toW/1 -> MinMax/2, Switch1/1
  pwrBW2Des/1 -> Switch/1
  ZeroPower/1 -> Switch/3
  Switch/1 -> MinMax/1
  Constant Power/1 -> kW_toW/1
  Discrete Transfer Fcn1/1 -> pwrBW2ActPhy/1

== stateflow chart Electrical_to_Thermal_gen/brakeResistor_with_delay_and_LPFilter/Inverter_State_Machine ==
  state Initialization
    en:
    BRC_ACT_InverterState = InvStInit;
    ActualValuesUpdate = 0;
  state Ready
    en:
    BRC_ACT_InverterState = InvStReady;
    ActualValuesUpdate = 1;
  state Error
    en:
    BRC_ACT_InverterState = InvStError;
    ActualValuesUpdate = 1;
  state Enable
    en:
    BRC_ACT_InverterState = InvStEnable;
    ActualValuesUpdate = 1;
  (default) -> Initialization
  Initialization -> Error [order 1] : [Error==1]
  Initialization -> Ready [order 2] : [Error==0]
  Error -> Ready : [BRC_CMD_Command == 4 &&  Error==0]
  Ready -> Error [order 2] : [Error==1]
  Enable -> Ready [order 1] : [BRC_CMD_Command == 0]
  Ready -> Enable [order 1] : [BRC_CMD_Command == 1]
  Enable -> Error [order 2] : [Error==1]
  data: BRC_CMD_Command input; BRC_ACT_InverterState output double; InvStEnable input; InvStError input; InvStReady input; InvStInit input; ActualValuesUpdate output double; Error input [0..1]

== stateflow chart Electrical_to_Thermal_gen/brakeResistor/Inverter_State_Machine ==
  state Initialization
    en:
    BRC_ACT_InverterState = InvStInit;
    ActualValuesUpdate = 0;
  state Ready
    en:
    BRC_ACT_InverterState = InvStReady;
    ActualValuesUpdate = 1;
  state Error
    en:
    BRC_ACT_InverterState = InvStError;
    ActualValuesUpdate = 1;
  state Enable
    en:
    BRC_ACT_InverterState = InvStEnable;
    ActualValuesUpdate = 1;
  (default) -> Initialization
  Initialization -> Error [order 1] : [Error==1]
  Initialization -> Ready [order 2] : [Error==0]
  Error -> Ready : [BRC_CMD_Command == 4 &&  Error==0]
  Ready -> Error [order 2] : [Error==1]
  Enable -> Ready [order 1] : [BRC_CMD_Command == 0]
  Ready -> Enable [order 1] : [BRC_CMD_Command == 1]
  Enable -> Error [order 2] : [Error==1]
  data: BRC_CMD_Command input; BRC_ACT_InverterState output double; InvStEnable input; InvStError input; InvStReady input; InvStInit input; ActualValuesUpdate output double; Error input [0..1]
